simulink model "sampleModel1406_2"  (R2023a)
settings: Solver=VariableStepAuto  StartTime=0.0  StopTime=10.0  RelTol=1e-3
libraries: hdlsllib x4
settings Model: Creator=user1  LastModifiedBy=user1

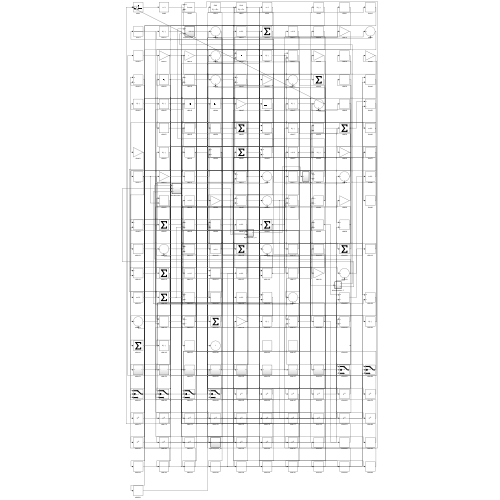
[thumbnail: Simulink's stored preview of the top-level diagram]
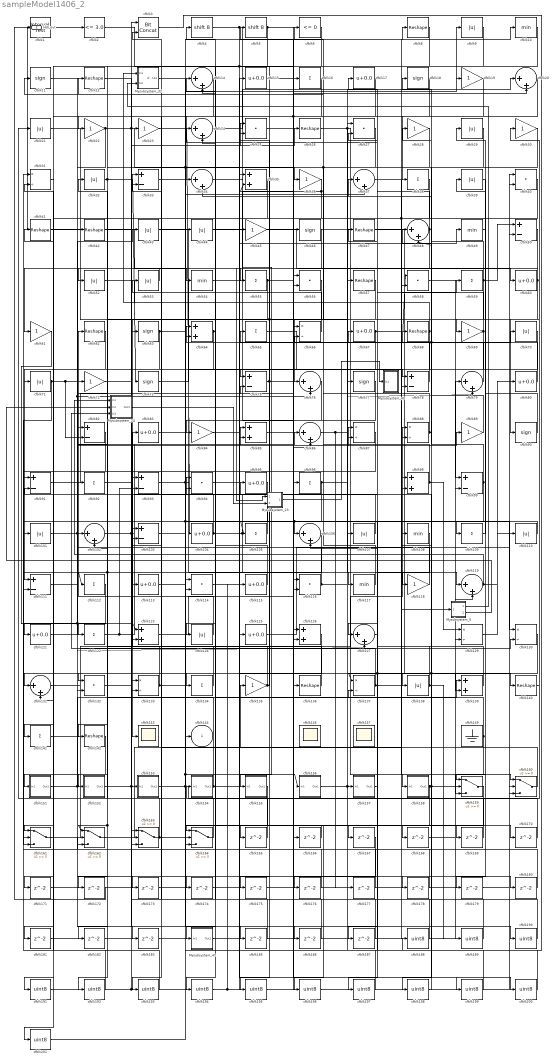
== system sampleModel1406_2 ==
  Mysubsystem_23 : Subsystem  TreatAsAtomicUnit=on  RTWFcnName=Mysubsystem_23
      settings: RTWFcnNameOpts=User specified  RTWFileNameOpts=Use function name
  Mysubsystem_24 : Subsystem  TreatAsAtomicUnit=on  RTWFcnName=Mysubsystem_24
      settings: RTWFcnNameOpts=User specified  RTWFileNameOpts=Use function name
  Mysubsystem_32 : Subsystem  TreatAsAtomicUnit=on  RTWFcnName=Mysubsystem_32
      settings: RTWFcnNameOpts=User specified  RTWFileNameOpts=Use function name
  Mysubsystem_40 : Subsystem  TreatAsAtomicUnit=on  RTWFcnName=Mysubsystem_40
      settings: RTWFcnNameOpts=User specified  RTWFileNameOpts=Use function name
  Mysubsystem_41 : Subsystem  TreatAsAtomicUnit=on  RTWFcnName=Mysubsystem_41
      settings: RTWFcnNameOpts=User specified  RTWFileNameOpts=Use function name
  Mysubsystem_5 : Subsystem  TreatAsAtomicUnit=on  RTWFcnName=Mysubsystem_5
      settings: RTWFcnNameOpts=User specified  RTWFileNameOpts=Use function name
  cfblk1 : hdlsllib/Logic and Bit Operations/Interval Test  IntervalClosedRight=on  uplimit=0.5  IntervalClosedLeft=on  lowlimit=-0.5  OutDataTypeStr=uint8
  cfblk{10,49,54,108,117} (5 alike) : MinMax  OutDataTypeStr=uint8
  cfblk{9,21,29,32,39,43..44,52..53,70..71,101,107,110,124,138} (16 alike) : Abs  OutDataTypeStr=uint8  SaturateOnIntegerOverflow=off
  cfblk{14,20,24,34,37,48,76,79,86,102,106,119,127,131} (14 alike) : Sum  Inputs=|++  OutDataTypeStr=uint8
  cfblk{33,50,75,78,82,91,93,99,103,111} (10 alike) : Sum  Inputs=+-  OutDataTypeStr=uint8
  cfblk{15,17,60,67,80,83,95,104,113,115,121,125} (12 alike) : Bias  Bias=0.0  SaturateOnIntegerOverflow=off
  cfblk{16,38,55,59,65,92,96,105,109,112,122,134,141} (13 alike) : Sum  Inputs=+  OutDataTypeStr=uint8
  cfblk{11,18,46,63,73,77,90} (7 alike) : Signum
  cfblk{25,27,40,56,58,94,114,116,132} (9 alike) : DotProduct  OutDataTypeStr=uint8
  cfblk{19,22..23,28,30,36,45,61,69,72,84,89,118,135} (14 alike) : Gain  OutDataTypeStr=uint8
  cfblk{8,12,26,41..42,47,57,62,68,136,140,142} (12 alike) : Reshape
  cfblk{35,64,85,98,123,126,139} (7 alike) : Sum  OutDataTypeStr=uint8
  cfblk{31,66,87..88,129..130,133,137} (8 alike) : Product  Inputs=*/  OutDataTypeStr=uint8  RndMeth=Zero  SaturateOnIntegerOverflow=on
  cfblk143 : Scope
  cfblk146 : Scope
      settings: Floating=on
  cfblk147 : Scope
      settings: Floating=on
  cfblk149 : Ground
  cfblk151 : Subsystem
      settings: LibrarySourceBlock=|
      | hdlsllib/Ports &
      | Subsystems/Subsystem
  cfblk152 : Subsystem
      settings: LibrarySourceBlock=|
      | hdlsllib/Ports &
      | Subsystems/Subsystem
  cfblk153 : Subsystem
      settings: LibrarySourceBlock=|
      | hdlsllib/Ports &
      | Subsystems/Subsystem
  cfblk154 : Subsystem
      settings: LibrarySourceBlock=|
      | hdlsllib/Ports &
      | Subsystems/Subsystem
  cfblk155 : Subsystem
      settings: LibrarySourceBlock=|
      | hdlsllib/Ports &
      | Subsystems/Subsystem
  cfblk156 : Subsystem
      settings: LibrarySourceBlock=|
      | hdlsllib/Ports &
      | Subsystems/Subsystem
  cfblk157 : Subsystem
      settings: LibrarySourceBlock=|
      | hdlsllib/Ports &
      | Subsystems/Subsystem
  cfblk158 : Subsystem
      settings: LibrarySourceBlock=|
      | hdlsllib/Ports &
      | Subsystems/Subsystem
  cfblk{159..164} (6 alike) : Switch  OutDataTypeStr=uint8  SaturateOnIntegerOverflow=off  InputSameDT=off
  cfblk{165..183,185..187} (22 alike) : Delay  SampleTime=1
  cfblk{188..201} (14 alike) : DataTypeConversion  OutDataTypeStr=uint8  SaturateOnIntegerOverflow=off  RndMeth=Floor
  cfblk2 : hdlsllib/Logic and Bit Operations/Compare To Constant  relop=<=  const=3.0  OutDataTypeStr=uint8
  cfblk3 : hdlsllib/Logic and Bit Operations/Bit Concat  numInputs=2
  cfblk4 : ArithShift  BitShiftNumber=8
  cfblk5 : ArithShift  BitShiftNumber=8
  cfblk6 : hdlsllib/Logic and Bit Operations/Compare To Zero  relop=<=  OutDataTypeStr=uint8
  cfblk144 : Outport  OutDataTypeStr=uint8  VectorParamsAs1DForOutWhenUnconnected=off
  Hdl_out : Outport  Port=2  OutDataTypeStr=uint8
  wires:
  cfblk55/1 -> cfblk143/1, cfblk20/2
  cfblk62/1 -> cfblk111/1
  cfblk1/1 -> cfblk2/1
  cfblk59/1 -> cfblk102/2, cfblk175/1, cfblk50/1, cfblk34/2
  cfblk135/1 -> cfblk61/1, cfblk64/2
  cfblk47/1 -> cfblk140/1
  cfblk80/1 -> cfblk58/1, cfblk48/2
  cfblk32/1 -> cfblk73/1, cfblk132/1
  cfblk61/1 -> cfblk122/1
  cfblk4/1 -> cfblk155/1(In1), cfblk139/2
  cfblk153/1(Out1) -> cfblk69/1, cfblk185/1
  cfblk129/1 -> cfblk110/1
  cfblk141/1 -> cfblk63/1
  cfblk138/1 -> cfblk95/1, cfblk189/1
  cfblk151/1(Out1) -> cfblk137/2, cfblk183/1
  cfblk98/1 -> cfblk129/1, cfblk11/1
  cfblk19/1 -> cfblk38/1
  cfblk9/1 -> cfblk91/1
  cfblk124/1 -> cfblk62/1
  cfblk26/1 -> cfblk158/1(In1), cfblk79/2
  cfblk58/1 -> cfblk99/1
  cfblk43/1 -> cfblk117/1
  cfblk21/1 -> cfblk76/1
  cfblk73/1 -> cfblk78/1
  cfblk64/1 -> cfblk133/1, cfblk134/1
  cfblk104/1 -> cfblk57/1, cfblk126/1, cfblk91/2
  cfblk56/1 -> cfblk112/1, cfblk172/1
  cfblk160/1 -> cfblk33/1
  cfblk29/1 -> cfblk36/1
  cfblk109/1 -> cfblk39/1
  cfblk118/1 -> cfblk102/1
  cfblk122/1 -> cfblk85/1, cfblk93/2
  cfblk16/1 -> cfblk104/1, cfblk116/2
  cfblk106/1 -> cfblk111/2
  cfblk110/1 -> cfblk106/1, cfblk105/1
  cfblk52/1 -> cfblk125/1
  cfblk34/1 -> cfblk136/1
  cfblk162/1 -> cfblk135/1
  cfblk105/1 -> cfblk83/1
  cfblk48/1 -> Mysubsystem_23/1(In1), cfblk24/1, Hdl_out/1
  cfblk41/1 -> cfblk42/1
  cfblk65/1 -> cfblk78/2
  cfblk116/1 -> cfblk4/1, cfblk20/1
  cfblk130/1 -> cfblk137/1, cfblk167/1, cfblk168/1
  cfblk156/1(Out1) -> cfblk157/1(In1), cfblk139/1
  cfblk93/1 -> cfblk130/1, cfblk6/1
  cfblk164/1 -> cfblk32/1
  cfblk78/1 -> cfblk67/1
  cfblk142/1 -> cfblk21/1
  cfblk87/1 -> cfblk141/1
  cfblk94/1 -> cfblk49/1
  cfblk133/1 -> cfblk44/1, cfblk92/1
  cfblk63/1 -> cfblk131/1, cfblk169/1
  cfblk83/1 -> cfblk156/1(In1), cfblk170/1
  cfblk158/1(Out1) -> cfblk159/2, cfblk98/2, cfblk195/1
  cfblk6/1 -> cfblk151/1(In1)
  cfblk46/1 -> cfblk133/2
  cfblk39/1 -> cfblk159/1
  cfblk136/1 -> cfblk72/1
  cfblk140/1 -> cfblk30/1
  cfblk132/1 -> cfblk87/1
  cfblk107/1 -> cfblk65/1
  cfblk68/1 -> Mysubsystem_32/1(In1), cfblk163/3
  cfblk44/1 -> cfblk107/1
  cfblk126/1 -> cfblk131/2
  cfblk5/1 -> cfblk22/1, cfblk178/1
  cfblk88/1 -> cfblk48/1, cfblk5/1
  cfblk95/1 -> cfblk164/2, cfblk123/2
  cfblk23/1 -> cfblk109/1
  cfblk75/1 -> cfblk138/1, cfblk25/2
  cfblk10/1 -> cfblk34/1
  cfblk149/1 -> cfblk94/1, cfblk159/3
  cfblk119/1 -> Mysubsystem_24/1(In1), cfblk80/1
  cfblk134/1 -> cfblk93/1
  cfblk111/1 -> cfblk87/2
  cfblk92/1 -> cfblk89/1
  cfblk121/1 -> cfblk86/1
  cfblk137/1 -> Mysubsystem_24/3(In3), cfblk10/1
  cfblk161/1 -> cfblk88/1
  cfblk33/1 -> cfblk26/1
  cfblk54/1 -> cfblk16/1
  cfblk89/1 -> cfblk28/1
  cfblk45/1 -> cfblk60/1
  cfblk50/1 -> cfblk142/1
  cfblk163/1 -> cfblk41/1, cfblk75/2
  cfblk69/1 -> cfblk164/3, cfblk17/1
  cfblk66/1 -> cfblk53/1
  cfblk99/1 -> cfblk18/1, cfblk127/1
  cfblk14/1 -> cfblk113/1
  cfblk115/1 -> cfblk14/1
  cfblk90/1 -> cfblk29/1
  cfblk152/1(Out1) -> cfblk68/1, cfblk190/1
  cfblk27/1 -> cfblk66/1, cfblk56/2
  cfblk2/1 -> cfblk45/1, cfblk46/1
  cfblk31/1 -> cfblk191/1
  cfblk123/1 -> cfblk86/2
  cfblk96/1 -> cfblk77/1, cfblk181/1
  cfblk18/1 -> cfblk152/1(In1)
  cfblk60/1 -> cfblk90/1, cfblk55/1
  cfblk17/1 -> cfblk121/1
  cfblk125/1 -> cfblk50/2
  cfblk24/1 -> cfblk9/1
  cfblk139/1 -> cfblk106/2
  cfblk70/1 -> cfblk101/1
  cfblk79/1 -> cfblk64/1
  cfblk42/1 -> cfblk54/1
  cfblk37/1 -> cfblk160/1
  cfblk53/1 -> cfblk52/1
  cfblk67/1 -> cfblk59/1, cfblk193/1
  cfblk91/1 -> cfblk8/1
  cfblk103/1 -> cfblk37/2
  cfblk22/1 -> cfblk94/2, cfblk96/1, cfblk180/1, cfblk132/2
  cfblk85/1 -> cfblk119/1
  cfblk35/1 -> cfblk162/1, cfblk192/1
  cfblk117/1 -> cfblk12/1
  cfblk20/1 -> cfblk84/1, cfblk126/2
  cfblk84/1 -> cfblk70/1
  cfblk131/1 -> cfblk130/2
  cfblk38/1 -> Mysubsystem_5/1(In1), cfblk161/1
  cfblk86/1 -> cfblk118/1, cfblk177/1
  cfblk102/1 -> cfblk98/1, cfblk174/1
  cfblk12/1 -> cfblk153/1(In1), cfblk186/1
  cfblk72/1 -> cfblk25/1
  cfblk57/1 -> cfblk103/1
  cfblk36/1 -> cfblk35/2, cfblk71/1
  cfblk8/1 -> cfblk75/1
  cfblk77/1 -> cfblk124/1
  cfblk157/1(Out1) -> cfblk47/1
  cfblk154/1(Out1) -> cfblk82/1, cfblk66/2
  cfblk40/1 -> cfblk194/1
  cfblk71/1 -> cfblk162/3, cfblk82/2, cfblk161/3
  cfblk113/1 -> cfblk19/1
  cfblk101/1 -> cfblk123/1, cfblk127/2, cfblk43/1, cfblk76/2
  cfblk76/1 -> cfblk165/1
  cfblk165/1 -> cfblk33/2
  cfblk25/1 -> cfblk166/1
  cfblk166/1 -> cfblk164/1
  cfblk168/1 -> cfblk119/2
  cfblk169/1 -> cfblk103/2
  cfblk170/1 -> cfblk24/2
  cfblk112/1 -> cfblk171/1
  cfblk171/1 -> cfblk129/2
  cfblk172/1 -> cfblk1/1
  cfblk11/1 -> cfblk173/1
  cfblk173/1 -> cfblk99/2
  cfblk174/1 -> cfblk58/2
  cfblk175/1 -> cfblk160/3
  cfblk159/1 -> cfblk176/1
  cfblk176/1 -> cfblk162/2
  cfblk177/1 -> cfblk14/2
  cfblk178/1 -> cfblk37/1
  cfblk49/1 -> cfblk179/1
  cfblk179/1 -> cfblk160/2
  cfblk180/1 -> cfblk161/2
  cfblk181/1 -> cfblk88/2
  cfblk28/1 -> cfblk182/1
  cfblk182/1 -> cfblk79/1
  cfblk183/1 -> cfblk35/1
  cfblk185/1 -> cfblk163/2
  cfblk186/1 -> cfblk163/1
  cfblk127/1 -> cfblk187/1
  cfblk187/1 -> cfblk116/1
  cfblk3/1 -> cfblk188/1
  cfblk188/1 -> cfblk154/1(In1)
  cfblk189/1 -> cfblk3/1
  cfblk190/1 -> cfblk3/2
  cfblk191/1 -> cfblk23/1, cfblk15/1
  cfblk192/1 -> cfblk31/1
  cfblk193/1 -> cfblk31/2
  cfblk194/1 -> cfblk56/1, cfblk115/1
  cfblk195/1 -> cfblk40/1
  cfblk167/1 -> cfblk196/1
  cfblk196/1 -> cfblk40/2
  cfblk108/1 -> cfblk197/1
  cfblk197/1 -> cfblk27/1
  cfblk30/1 -> cfblk198/1
  cfblk198/1 -> cfblk108/1
  cfblk114/1 -> cfblk199/1
  cfblk199/1 -> cfblk27/2
  cfblk15/1 -> cfblk200/1
  cfblk200/1 -> cfblk114/1
  cfblk82/1 -> cfblk201/1
  cfblk201/1 -> cfblk114/2
  Mysubsystem_5/2(Out2) -> Mysubsystem_24/2(In2)
  Mysubsystem_24/1(Out1) -> Mysubsystem_23/2(In2)
  Mysubsystem_5/1(Out1) -> Mysubsystem_32/2(In2)
  Mysubsystem_32/1(cfblk144) -> cfblk144/1
  Mysubsystem_23/1(Out1) -> Mysubsystem_40/1(In1)
  cfblk155/1(Out1) -> Mysubsystem_41/1(In1)
  Mysubsystem_41/1(Out1) -> cfblk85/2

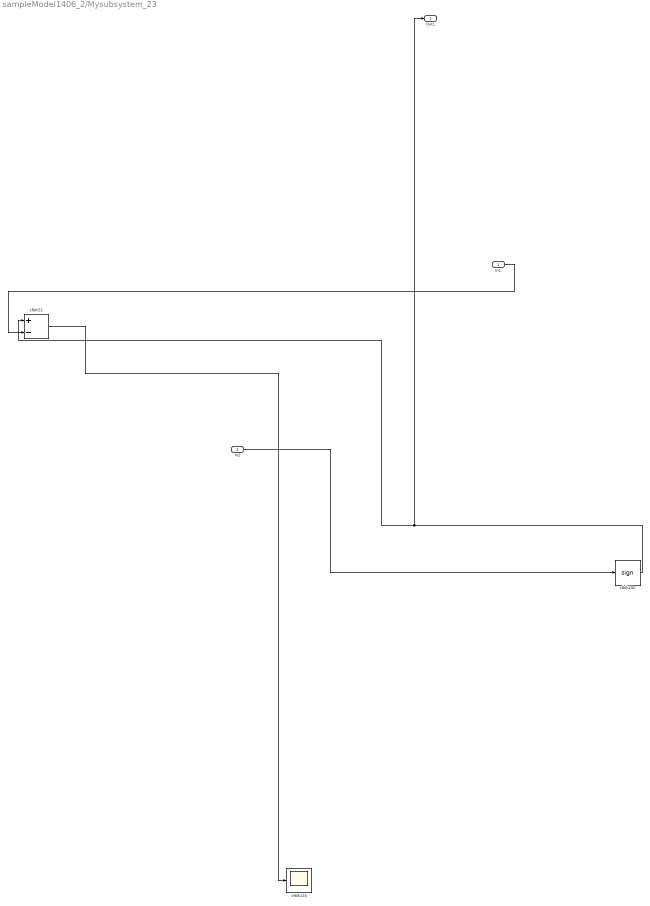
== system sampleModel1406_2/Mysubsystem_23 ==
  In1 : Inport
  In2 : Inport  Port=2
  cfblk100 : Signum
  cfblk145 : Scope
  cfblk51 : Sum  Inputs=+-
  Out1 : Outport
  wires:
  cfblk51/1 -> cfblk145/1
  In2/1 -> cfblk100/1
  cfblk100/1 -> Out1/1, cfblk51/1
  In1/1 -> cfblk51/2

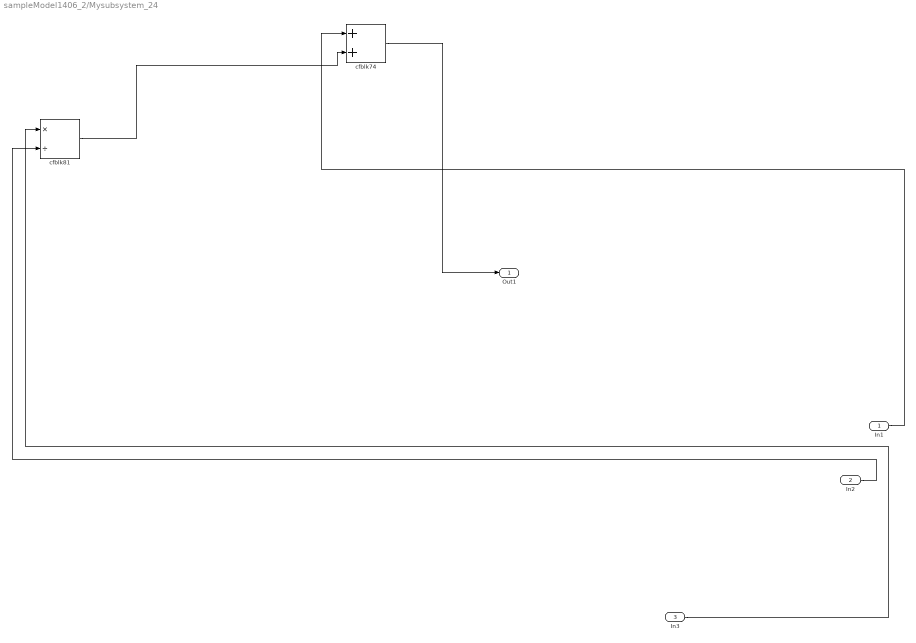
== system sampleModel1406_2/Mysubsystem_24 ==
  In1 : Inport
  In2 : Inport  Port=2
  In3 : Inport  Port=3
  cfblk74 : Sum
  cfblk81 : Product  Inputs=*/  RndMeth=Zero  SaturateOnIntegerOverflow=on
  Out1 : Outport
  wires:
  cfblk81/1 -> cfblk74/2
  In1/1 -> cfblk74/1
  In3/1 -> cfblk81/1
  cfblk74/1 -> Out1/1
  In2/1 -> cfblk81/2

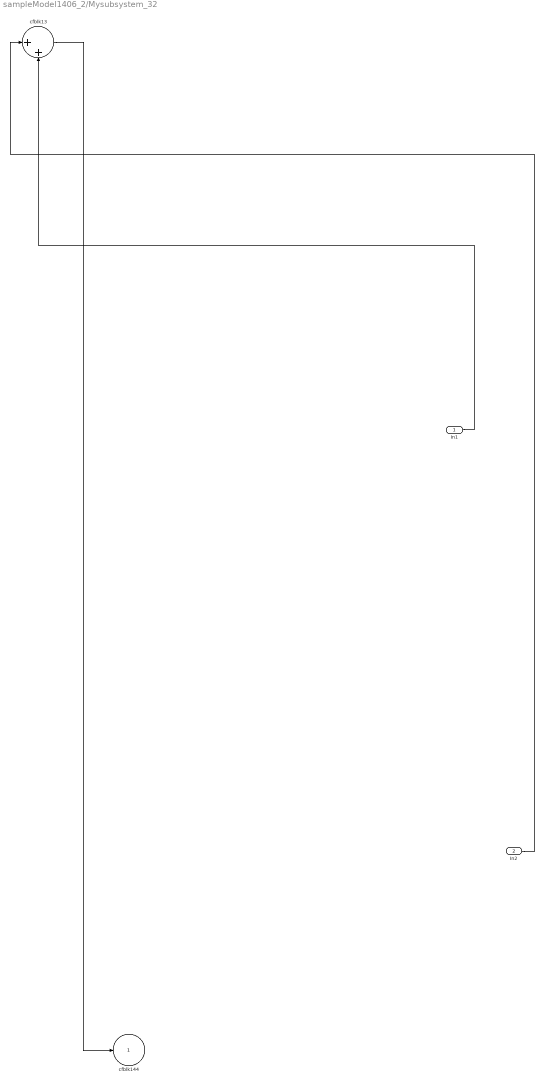
== system sampleModel1406_2/Mysubsystem_32 ==
  In1 : Inport
  In2 : Inport  Port=2
  cfblk13 : Sum  Inputs=|++
  cfblk144 : Outport  VectorParamsAs1DForOutWhenUnconnected=off
  wires:
  cfblk13/1 -> cfblk144/1
  In1/1 -> cfblk13/2
  In2/1 -> cfblk13/1

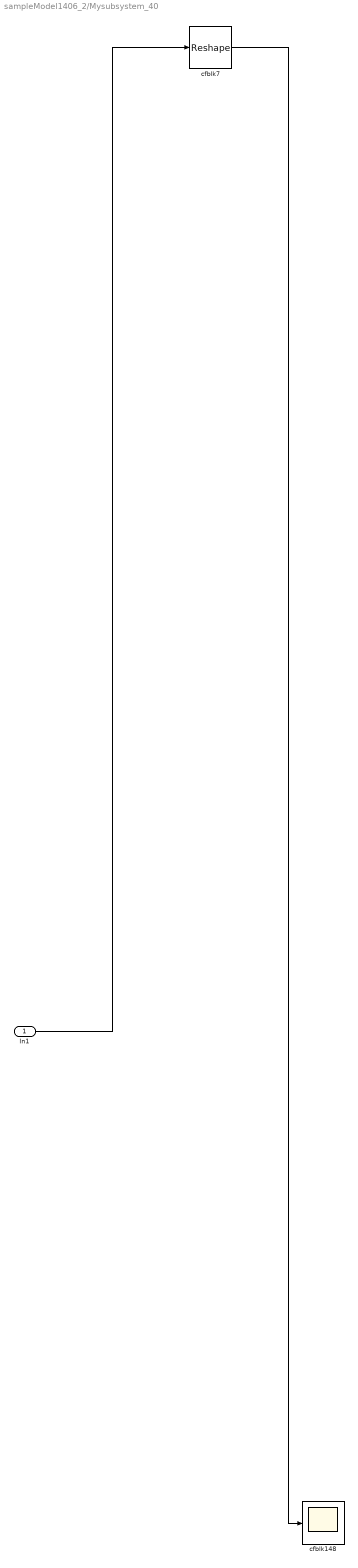
== system sampleModel1406_2/Mysubsystem_40 ==
  In1 : Inport
  cfblk148 : Scope
  cfblk7 : Reshape
  wires:
  In1/1 -> cfblk7/1
  cfblk7/1 -> cfblk148/1

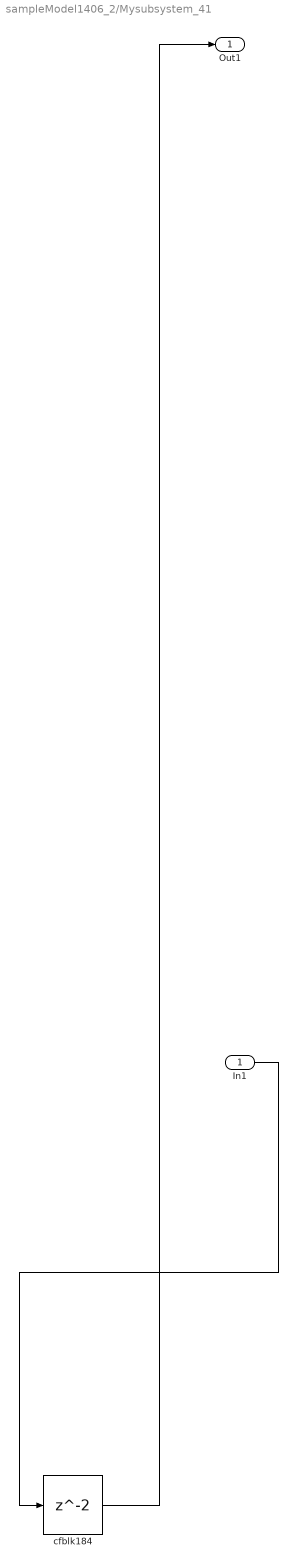
== system sampleModel1406_2/Mysubsystem_41 ==
  In1 : Inport
  cfblk184 : Delay  SampleTime=1
  Out1 : Outport
  wires:
  cfblk184/1 -> Out1/1
  In1/1 -> cfblk184/1

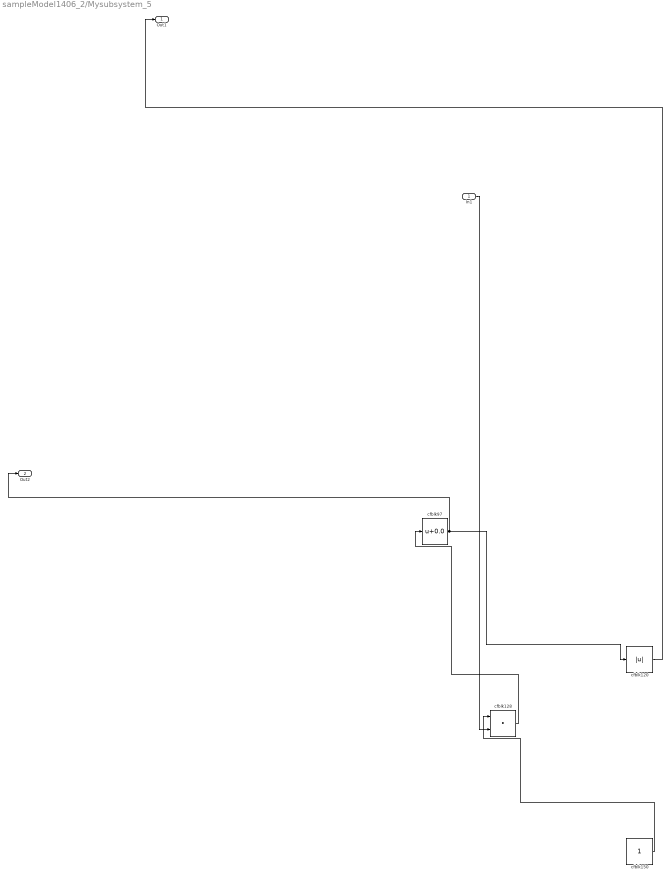
== system sampleModel1406_2/Mysubsystem_5 ==
  In1 : Inport
  cfblk120 : Abs  SaturateOnIntegerOverflow=off
  cfblk128 : DotProduct  OutDataTypeStr=Inherit: Inherit via internal rule
  cfblk150 : Constant  SampleTime=-1
  cfblk97 : Bias  Bias=0.0  SaturateOnIntegerOverflow=off
  Out1 : Outport
  Out2 : Outport  Port=2
  wires:
  cfblk150/1 -> cfblk128/1
  cfblk97/1 -> Out2/1, cfblk120/1
  cfblk120/1 -> Out1/1
  In1/1 -> cfblk128/2
  cfblk128/1 -> cfblk97/1

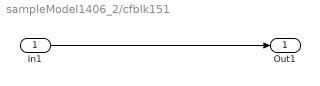
== system sampleModel1406_2/cfblk151 ==
  In1 : Inport
  Out1 : Outport
  wires:
  In1/1 -> Out1/1

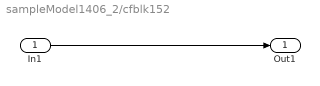
== system sampleModel1406_2/cfblk152 ==
  In1 : Inport
  Out1 : Outport
  wires:
  In1/1 -> Out1/1

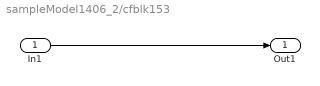
== system sampleModel1406_2/cfblk153 ==
  In1 : Inport
  Out1 : Outport
  wires:
  In1/1 -> Out1/1

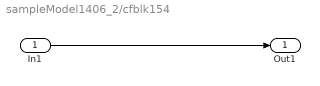
== system sampleModel1406_2/cfblk154 ==
  In1 : Inport
  Out1 : Outport
  wires:
  In1/1 -> Out1/1

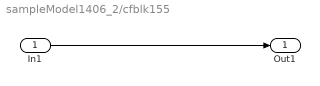
== system sampleModel1406_2/cfblk155 ==
  In1 : Inport
  Out1 : Outport
  wires:
  In1/1 -> Out1/1

== system sampleModel1406_2/cfblk156 ==
  In1 : Inport
  Out1 : Outport
  wires:
  In1/1 -> Out1/1

== system sampleModel1406_2/cfblk157 ==
  In1 : Inport
  Out1 : Outport
  wires:
  In1/1 -> Out1/1

== system sampleModel1406_2/cfblk158 ==
  In1 : Inport
  Out1 : Outport
  wires:
  In1/1 -> Out1/1
